simulink model "L0503"  (Simulink 9.1)
settings: Solver=VariableStepDiscrete  StartTime=0.0  StopTime=inf  MaxStep=0.1  RelTol=1e-3
settings Model: Creator=Asus  LastModifiedBy=Asus
settings DataIOCC: SaveFormat=Dataset
settings OptimizationCC: LifeSpan=auto
settings DebuggingCC: UnderspecifiedInitializationDetection=Simplified  MergeDetectMultiDrivingBlocksExec=error  SFUnexpectedBacktrackingDiag=error  SFNoUnconditionalDefaultTransitionDiag=error  SFExecutionAtInitializationDiag=warning
settings HardwareCC: ProdBitPerPointer=64  ProdBitPerSizeT=64  ProdBitPerPtrDiffT=64  ProdLargestAtomicFloat=Float  ProdIntDivRoundTo=Zero  ProdEndianess=LittleEndian  ProdWordSize=64  ProdHWDeviceType=Intel->x86-64 (Windows64)
settings ModelReferenceCC: PropagateSignalLabelsOutOfModel=on
settings CodeAppCC: StateflowObjectComments=off
settings GRTTargetCC: TargetLangStandard=C99 (ISO)  CombineOutputUpdateFcns=on  GRTInterface=off
settings ConfigComp: CovMetricSettings=dwe  CovHtmlReporting=off  CovSaveCumulativeToWorkspaceVar=off  CovSaveSingleToWorkspaceVar=off  CovExternalEMLEnable=on

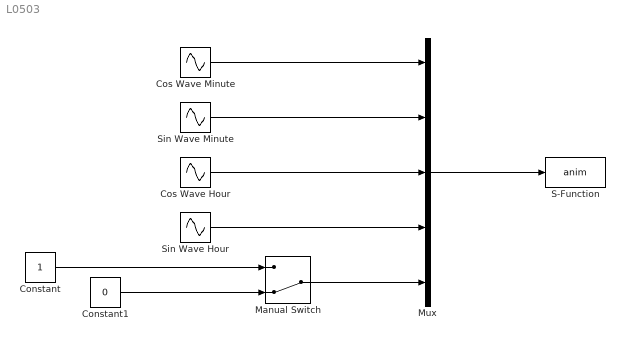
== system L0503 ==
  Constant : Constant
  Constant1 : Constant  Value=0
  Cos Wave Hour : Sin  Frequency=pi/360  Phase=pi/2  SampleTime=0
  Cos Wave Minute : Sin  Frequency=pi/30  Phase=pi/2  SampleTime=0
  Manual Switch : ManualSwitch  CurrentSetting=0
  Mux : Mux  Inputs=5
  S-Function : S-Function  FunctionName=anim  Parameters=0.1  SFunctionDeploymentMode=off  EnableBusSupport=off
  Sin Wave Hour : Sin  Frequency=pi/360  SampleTime=0
  Sin Wave Minute : Sin  Frequency=pi/30  SampleTime=0
  wires:
  Cos Wave Minute/1 -> Mux/1
  Sin Wave Minute/1 -> Mux/2
  Cos Wave Hour/1 -> Mux/3
  Sin Wave Hour/1 -> Mux/4
  Mux/1 -> S-Function/1
  Constant/1 -> Manual Switch/1
  Constant1/1 -> Manual Switch/2
  Manual Switch/1 -> Mux/5
